simulink model "lateralControl"  (R2019a)
settings: Solver=ode45  StartTime=0.0  StopTime=20  RelTol=1e-3
undefined symbols (not defined in the file): C_af, C_ar, g, Iz, lf, lr, m, sigbuilder_block
libraries: simulink x2
settings Model: DataDictionary=VehicleData.sldd  Creator=headl  LastModifiedBy=headl
settings DataIOCC: ReturnWorkspaceOutputs=off  DSMLoggingName=datalog
settings DebuggingCC: SignalRangeChecking=warning

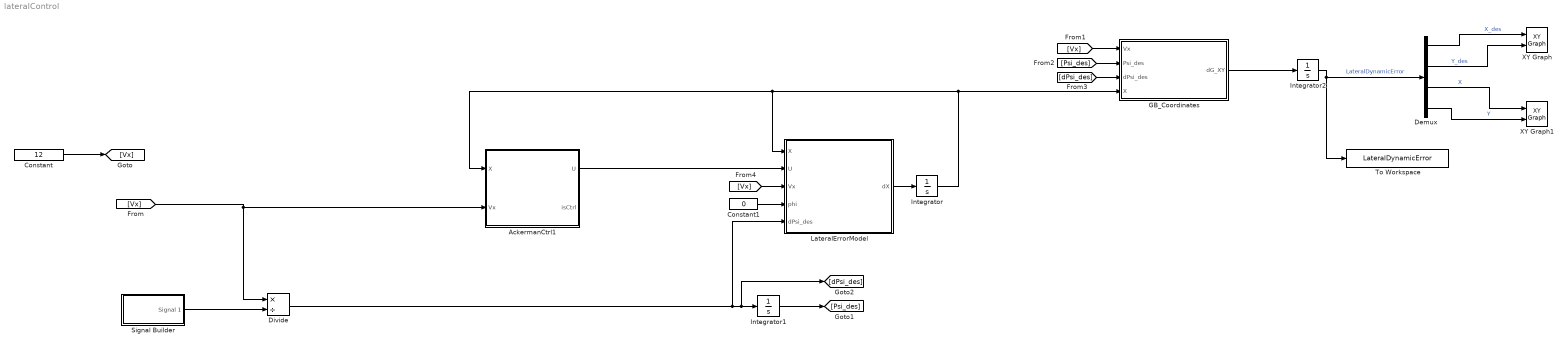
== system lateralControl ==
  AckermanCtrl1 : MATLAB Function  TreatAsAtomicUnit=on
  Constant : Constant  Value=12
  Constant1 : Constant  Value=0
  Demux : Demux
  Divide : Product  Inputs=*/
  GB_Coordinates : MATLAB Function  TreatAsAtomicUnit=on
  Integrator : Integrator  InitialCondition=[1;1;1;1]
  Integrator1 : Integrator
  Integrator2 : Integrator  InitialCondition=[0;0;0;0]
  LateralErrorModel : MATLAB Function  TreatAsAtomicUnit=on
  Signal Builder : Subsystem  Tag=STV Subsys  LoadFcn=sigbuilder_block('load');  StartFcn=sigbuilder_block('start');  StopFcn=sigbuilder_block('stop');  ClipboardFcn=sigbuilder_block('clipboard');  mask(Sigbuilder block){tuvar=[0:10]}
      mask help: Simulink:masks:SigbuilderBlock_MD
      mask init:
      | if ~strcmp(get_param(bdroot(gcbh),'SimulationStatus'),'stopped') tuvar = sigbuilder_block('maskInit'); end
      settings: CopyFcn=sigbuilder_block('copy');  DeleteFcn=sigbuilder_block('delete');  ModelCloseFcn=sigbuilder_block('modelClose');  PreSaveFcn=sigbuilder_block('preSave');  PauseFcn=sigbuilder_block('pause');  ContinueFcn=sigbuilder_block('continue');  NameChangeFcn=sigbuilder_block('namechange');  OpenFcn=sigbuilder_block('open',[437.6 199.2 550.4 400 ]);  CloseFcn=sigbuilder_block('close');
      mask Display: plot(0, 0, 100, 100,[2, 2, 32, 32, 2], [68, 8, 8, 68, 68],[32, 2], [38, 38], [32, 19, 2],[53, 60, 44], [32, 17, 17, 2],[16, 16, 31, 31]);txt = getActiveGroup(gcbh);text(2, 100, txt,'verticalAlignment', 'top');
  To Workspace : ToWorkspace  VariableName=LateralDynamicError  SampleTime=-1
  XY Graph : simulink/Sinks/XY Graph  xmin=-20  xmax=100  ymin=-20  ymax=100  st=-1
  XY Graph1 : simulink/Sinks/XY Graph  xmin=-20  xmax=100  ymin=-20  ymax=100  st=-1
  wires:
  LateralErrorModel/1(dX) -> Integrator/1
  Integrator/1 -> GB_Coordinates/4(X), AckermanCtrl1/1(X), LateralErrorModel/1(X)
  Constant1/1 -> LateralErrorModel/4(phi)
  Signal Builder/1(Signal 1) -> Divide/2
  GB_Coordinates/1(dG_XY) -> Integrator2/1
  [Vx] -> AckermanCtrl1/2(Vx), Divide/1
  Constant/1 -> [Vx]
  [Vx] -> GB_Coordinates/1(Vx)
  Divide/1 -> LateralErrorModel/5(dPsi_des), [dPsi_des], Integrator1/1
  Integrator1/1 -> [Psi_des]
  [Psi_des] -> GB_Coordinates/2(Psi_des)
  [dPsi_des] -> GB_Coordinates/3(dPsi_des)
  Integrator2/1 -> To Workspace/1, Demux/1  "LateralDynamicError"
  Demux/1 -> XY Graph/1  "X_des"
  Demux/2 -> XY Graph/2  "Y_des"
  Demux/3 -> XY Graph1/1  "X"
  Demux/4 -> XY Graph1/2  "Y"
  [Vx] -> LateralErrorModel/3(Vx)
  AckermanCtrl1/1(U) -> LateralErrorModel/2(U)

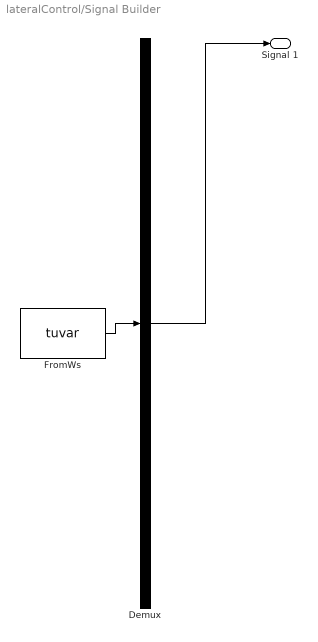
== system lateralControl/Signal Builder ==
  Demux : Demux  Tag=STV Demux  Outputs=1
  FromWs : FromWorkspace  Tag=STV FromWs  VariableName=tuvar  SampleTime=0
      SigBuilderData=|
      | common.afterFinalStr = 'Extrapolate'
      | common.sampleTime = 0
      | dataSet.timeRange = [0 20]
      | dataSet.name = 'Group 1'
      | sbobj.Groups.Name = 'Group 1'
      | sbobj.Groups.Signals.Name = 'Signal 1'
      | sbobj.Groups.Signals.XData = [0 5 5 10 10 15 15 20]
      | sbobj.Groups.Signals.YData = [50 50 -50 -50 50 50 -50 -50]
      | sbobj.Groups.TimeRange = [0 20]
  Signal 1 : Outport  Tag=STV Outport
  wires:
  Demux/1 -> Signal 1/1
  FromWs/1 -> Demux/1

== matlab function lateralControl/LateralErrorModel ==
  data: X input; dX output; U input; Vx input; phi input; dPsi_des input; g parameter; C_af parameter; C_ar parameter; lf parameter; lr parameter; Iz parameter; m parameter
% ******************* Lateral dynamic model of error *****************
%*********************************************************************
% Author: L.Arturo Torres-Romero
% Date: 22-10-2020
% This controller controlls the direction of a car, based in the dynamics
% described  in the next link and using the Ackerman formulation: 
% https://www.researchgate.net/publication/340166902_LATERAL_VEHICLE_DYNAMICS_AND_CONTROLLERS_DESIGN


%******************* PARAMETERS DESCRIPTIONS **********************
%******************************************************************
% m: vehicle mass
% g: gravity
% C_af : Cornering  stiffness  of  front  wheels.
% C_ar : Cornering  stiffness  of  rear  wheels.
% lf : distance fron the center of gravity to the front wheel axis.
% lr : distance fron the center of gravity to the rear wheel axis.
% Iz : this is the momentum of inertia of the vehicle respect the z axis.
%******************************************************************
%******************* INPUTS DESCRIPTIONS **************************
%******************************************************************
% X:   (column vector)[e1;de1;e2;de2] states of the state space of 
%       the system that includes the errors as follows:
%      e1  : is the lateral position error respect the road.
%      de1 : derivative of e1.
%      e2  : is the yaw angle error with respect the road. 
%      de2 : derivarive of the e2.

% U: (rad) angle in radians of the front wheel respect to longitudinal
%     vehicle axis
% Vx: (m/s) Logitudinal velocity.
% phi: (rad)inclination of the road.
% dPsi_des: (rad/s)angular velocity of the yaw. (orientation of the car.


%******************************************************************
% ******************* OUTPUTS DESCRIPTIONS ************************
%******************************************************************
% dX: derivative of X.
%******************************************************************

function dX = lateralErrorModel(X,U,Vx,phi,dPsi_des, g, C_af, C_ar, lf, lr, Iz, m)
dX = [0;0;0;0];
e1 =  X(1);
de1 = X(2);
e2 =  X(3);
de2 = X(4);

%**************************************************
%******* Matrix A formulation *********************
A22 = -(2*C_af + 2*C_ar)/(m*Vx);
A23 = (2*C_af + 2*C_ar)/m;
A24 = (-2*C_af*lf + 2*C_ar*lr)/(m*Vx);
A42 = -(2*C_af*lf - 2*C_ar*lr)/(Iz*Vx);
A43 = (2*C_af*lf - 2*C_ar*lr)/Iz;
A44 = -(2*C_af*lf^2 + 2*C_ar*lr^2)/(Iz*Vx);

A = [0 1 0 0;0 A22 A23 A24;0 0 0 1;0 A42 A43 A44];
%**************************************************

%**************************************************
%******* Matrix B1 formulation ********************
B1_2 = 2*C_af/m;
B1_4 = 2*C_af*lf/Iz;

B1 = [0;B1_2;0;B1_4];
%***************************************************

%***************************************************
%******* Matrix B2 formulation *********************
B2_2 = -(2*C_af*lf - 2*C_ar*lr)/(m*Vx) - Vx;
B2_4 = -(2*C_af*lf^2 + 2*C_ar*lr^2)/(Iz*Vx);

B2 = [0;B2_2;0;B2_4];
%***************************************************


%***************************************************
%******* Matrix B3 formulation *********************
B3 = [0;g;0;0];
%***************************************************


dX = A*X + B1*U + B2*dPsi_des + B3*sin(phi);

== matlab function lateralControl/GB_Coordinates ==
  data: Vx input; dG_XY output; Psi_des input; dPsi_des input; X input
function dG_XY = GB_Coordinates(Vx,Psi_des,dPsi_des,X)
dG_XY = [0;0;0;0];
e1 = X(1);
de1 = X(2);
e2 = X(3);
de2 = X(4);

%Global Coordinates calculation
%V = sqrt(Vx^2+de1^2);
G_dX_des = Vx*cos(Psi_des);
G_dY_des = Vx*sin(Psi_des);
G_dX = G_dX_des  - (de1*sin(e2 + Psi_des ) + e1*cos(e2 + Psi_des)*(de2 + dPsi_des));
G_dY = G_dY_des  + (de1*cos(e2 + Psi_des ) - e1*sin(e2 + Psi_des)*(de2 + dPsi_des));


dG_XY(1) = G_dX_des;
dG_XY(2) = G_dY_des;
dG_XY(3) = G_dX;
dG_XY(4) = G_dY;

== matlab function lateralControl/AckermanCtrl1 ==
  data: U output size=1; X input; Vx input; isCtrl output; C_af parameter; g parameter; C_ar parameter; lf parameter; lr parameter; Iz parameter; m parameter
% ******************* Lateral dynamic controller *********************
%*********************************************************************
% Author: L.Arturo Torres-Romero
% Date: 22-10-2020
% This controller controlls the direction of a car, based in the dynamics
% described  in the next link and using the Ackerman formulation: 
% https://www.researchgate.net/publication/340166902_LATERAL_VEHICLE_DYNAMICS_AND_CONTROLLERS_DESIGN


%******************* PARAMETERS DESCRIPTIONS **********************
%******************************************************************
% m: vehicle mass
% g: gravity
% C_af : Cornering  stiffness  of  front  wheels.
% C_ar : Cornering  stiffness  of  rear  wheels.
% lf : distance fron the center of gravity to the front wheel axis.
% lr : distance fron the center of gravity to the rear wheel axis.
% Iz : this is the momentum of inertia of the vehicle respect the z axis.
%******************************************************************
%******************* INPUTS DESCRIPTIONS **************************
%******************************************************************
% X:   (column vector)[e1;de1;e2;de2] states of the state space of 
%       the system that includes the errors as follows:
%      e1  : is the lateral position error respect the road.
%      de1 : derivative of e1.
%      e2  : is the yaw angle error with respect the road. 
%      de2 : derivarive of the e2.

% Vx: Logitudinal velocity.



%******************************************************************
% ******************* OUTPUTS DESCRIPTIONS ************************
%******************************************************************
% U: control coutput in radians. Angle of the frontal wheels respect to the
%    longitudinal axis
% isCtrl: when true means that the matrix Mc has full rank, and hence, the
%         system is controllable


%******************************************************************


function [U,isCtrl] = AckermanLateralCtrl(X, Vx, C_af, g, C_ar, lf, lr, Iz, m) % pd polos deseados

%**************************************************
%******* Matrix A formulation *********************
A22 = -(2*C_af + 2*C_ar)/(m*Vx);
A23 = (2*C_af + 2*C_ar)/m;
A24 = (-2*C_af*lf + 2*C_ar*lr)/(m*Vx);
A42 = -(2*C_af*lf - 2*C_ar*lr)/(Iz*Vx);
A43 = (2*C_af*lf - 2*C_ar*lr)/Iz;
A44 = -(2*C_af*lf^2 + 2*C_ar*lr^2)/(Iz*Vx);

A = [0 1 0 0;0 A22 A23 A24;0 0 0 1;0 A42 A43 A44];
%**************************************************

%**************************************************
%******* Matrix B1 formulation ********************
B1_2 = 2*C_af/m;
B1_4 = 2*C_af*lf/Iz;

B1 = [0;B1_2;0;B1_4];
%***************************************************

%***************************************************
%******* Matrix B2 formulation *********************
B2_2 = -(2*C_af*lf - 2*C_ar*lr)/(m*Vx) - Vx;
B2_4 = -(2*C_af*lf^2 + 2*C_ar*lr^2)/(Iz*Vx);

B2 = [0;B2_2;0;B2_4];
%***************************************************


%***************************************************
%******* Matrix B3 formulation *********************
B3 = [0;g;0;0];
%***************************************************


%***************************************************
%******* Verification of controllability and output 
% calculation of the controller
%**************************************************
ctrlVal = 0;
Mc = [B1 A*B1 A^2*B1 A^3*B1];
rankVal = rank(Mc);
    if rankVal < size(A,1)
        %disp('Not completely state controllable');
        isCtrl = 0;
        ctrlVal = 0;
    else
        %disp('Completely state controllable');
        isCtrl = 1;
        % Pole placement
        Pd =[-5-3i -5+3i -7 -10];
        %Pd =[-2 -2 -2 -2];

        H = (A- Pd(1)*eye(4)) * (A- Pd(2)*eye(4)) * (A- Pd(3)*eye(4)) * (A- Pd(4)*eye(4));

        %ackerman formula
        K = [0 0 0 1]*Mc^-1*H;
        ctrlVal = -K*X;  
    end


U = real(ctrlVal);
